simulink model "Leadcomp"  (R2023a)
settings: Solver=VariableStepAuto  StartTime=0.0  StopTime=10  RelTol=1e-3
undefined symbols (not defined in the file): N4
settings Model: Creator=velid  LastModifiedBy=velid

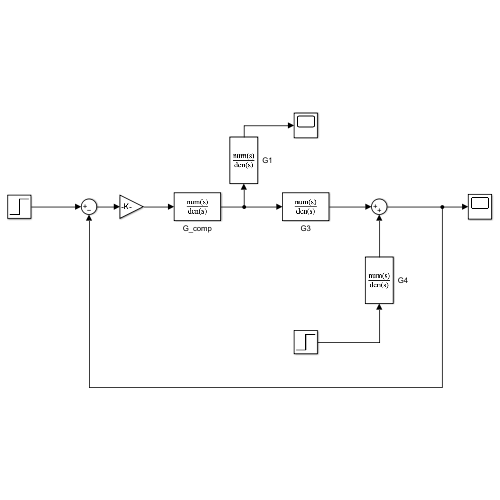
[thumbnail: Simulink's stored preview of the top-level diagram]
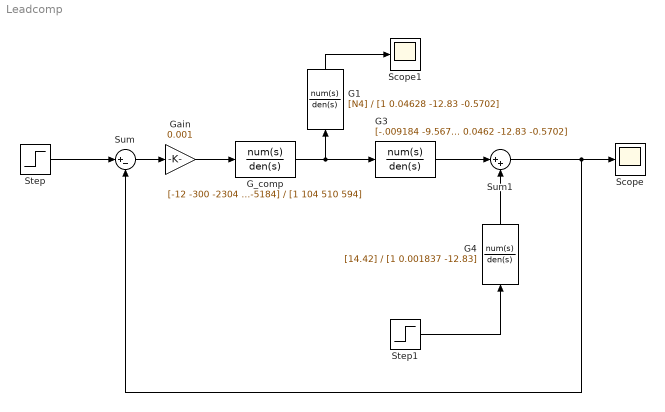
== system Leadcomp ==
  G1 : TransferFcn  Numerator=[N4]  Denominator=[1 0.04628 -12.83 -0.5702]
  G3 : TransferFcn  Numerator=[-.009184 -9.5673e-06]  Denominator=[1 0.0462 -12.83 -0.5702]
  G4 : TransferFcn  Numerator=[14.42]  Denominator=[1 0.001837 -12.83]
  G_comp : TransferFcn  Numerator=[-12 -300 -2304 -5184]  Denominator=[1 104 510 594]
  Gain : Gain  Gain=0.001
  Scope : Scope
  Scope1 : Scope
  Step : Step  SampleTime=0
  Step1 : Step  SampleTime=0
  Sum : Sum  Inputs=|+-
  Sum1 : Sum  Inputs=|++
  wires:
  G_comp/1 -> G1/1, G3/1
  Step/1 -> Sum/1
  Sum/1 -> Gain/1
  G3/1 -> Sum1/1
  G4/1 -> Sum1/2
  Step1/1 -> G4/1
  Sum1/1 -> Sum/2, Scope/1
  Gain/1 -> G_comp/1
  G1/1 -> Scope1/1
